simulink model "WaterTank"  (R2023b)
settings: Solver=VariableStepAuto  StartTime=0.0  StopTime=10.0  RelTol=1e-3
undefined symbols (not defined in the file or in its folder): h0
libraries: mci_models x1
settings Model: Creator=12064  LastModifiedBy=12064

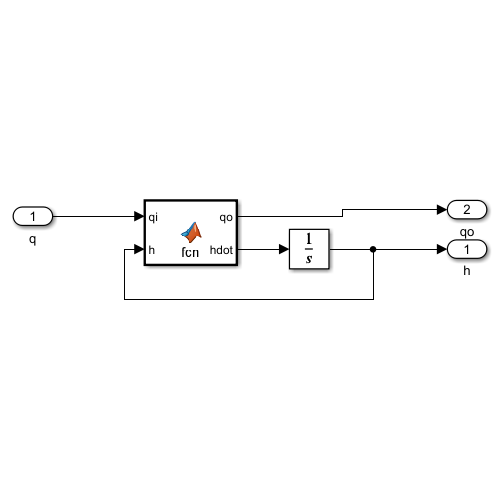
[thumbnail: Simulink's stored preview of the top-level diagram]
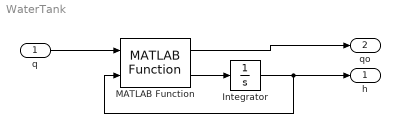
== system WaterTank ==
  q : Inport
  Integrator : Integrator  InitialCondition=h0
  MATLAB Function : mci_models/Fluid Systems/Tank with Outflow/MATLAB Function  SystemSampleTime=-1  VariantActivationTime=update diagram  AllowFlexibleInterface=on  Latency=0  AutoFrameSizeCalculation=off
  h : Outport  VectorParamsAs1DForOutWhenUnconnected=off
  qo : Outport  Port=2  VectorParamsAs1DForOutWhenUnconnected=off
  wires:
  MATLAB Function/1 -> qo/1
  Integrator/1 -> h/1, MATLAB Function/2
  MATLAB Function/2 -> Integrator/1
  q/1 -> MATLAB Function/1
